simulink model "LQI"  (R2024a)
settings: Solver=VariableStepAuto  StartTime=0.0  StopTime=2.5  RelTol=1e-3
values from neighbouring files (symbols this model uses):
  A = [A11 A12 A13 A14; A21 A22 A23 A24; A31 A32 A33 A34; A41 A42 A43 A44]    [FurutaLineal.m]    (also in ModeloFuruta.m = [0      0       1       0)
  B = [B11 B12; B21 B22; B31 B32; B41 B42]    [FurutaLineal.m]    (also in ModeloFuruta.m = [0)
  D = [2*I_x*block.ContStates.Data(4)*cos(block.ContStates.Data(2))*sin(block.ContStates.Data(2)), -C_z*M_2*l_bi*sin(block.ContStates.Data(2))*block.ContStates.Data(4); -I_x*block.ContStates.Data(3)*cos(block.ContStates.Data(2))*sin(block.ContStates.Data(2)), 0]    [FurutanolinealSLV2.m]
  K = 1.29    [FurutanolinealSLV2.m]
undefined symbols (not defined in the file or in its folder): A1, B1, C, C1, D1, K1
settings Model: Creator=PC  LastModifiedBy=PC
settings SolverCC: MaxConsecutiveMinStep=100
settings RTWCC: GPUComputeCapability=3.5

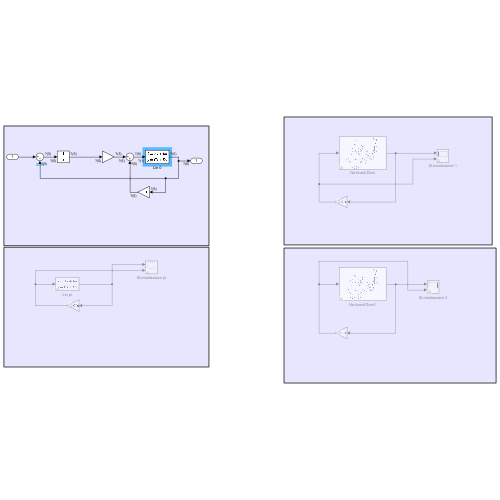
[thumbnail: Simulink's stored preview of the top-level diagram]
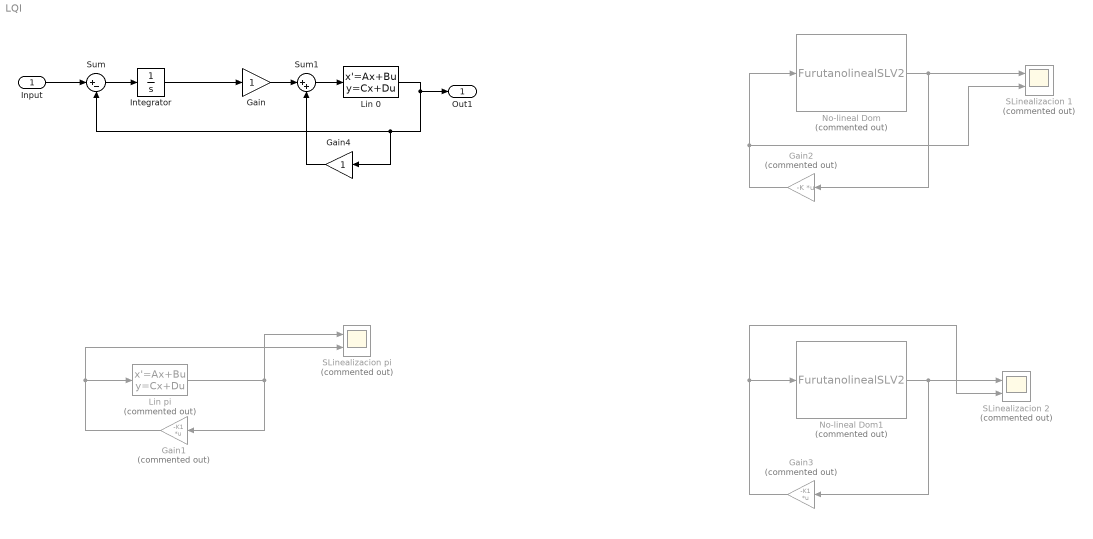
== system LQI ==
  Input : Inport
  Gain : Gain
  Gain1 : Gain  Commented=on  Gain=-K1  Multiplication=Matrix(K*u)
  Gain2 : Gain  Commented=on  Gain=-K  Multiplication=Matrix(K*u)
  Gain3 : Gain  Commented=on  Gain=-K1  Multiplication=Matrix(K*u)
  Gain4 : Gain
  Integrator : Integrator
  Lin 0 : StateSpace  A=A  B=B  C=C  D=D  InitialCondition=[0;0;0;0;0]  ParameterTunability=Unconstrained  AllowTunableDMatrix=on
  Lin pi : StateSpace  Commented=on  A=A1  B=B1  C=C1  D=D1  InitialCondition=[0;pi;0;0;0]  ParameterTunability=Unconstrained  AllowTunableDMatrix=on
  No-lineal Dom : M-S-Function  Commented=on  FunctionName=FurutanolinealSLV2  mask{Xi=0, g=0, J=0, M_2=0, l_bi=0, C_x=0, C_z=0, I_x=0, I_z=0}
      mask prompts: Xi "Parametros iniciales (Xi)"
      mask Display: image('mascara2.png');
  No-lineal Dom1 : M-S-Function  Commented=on  FunctionName=FurutanolinealSLV2  mask{Xi=0, g=0, J=0, M_2=0, l_bi=0, C_x=0, C_z=0, I_x=0, I_z=0}
      mask prompts: Xi "Parametros iniciales (Xi)"
      mask Display: image('mascara2.png');
  SLinealizacion 1 : Scope  Commented=on  NumInputPorts=2
  SLinealizacion 2 : Scope  Commented=on  NumInputPorts=2
  SLinealizacion pi : Scope  Commented=on  NumInputPorts=2
  Sum : Sum  Inputs=|+-
  Sum1 : Sum  Inputs=|++
  Out1 : Outport
  wires:
  Lin pi/1 -> Gain1/1, SLinealizacion pi/1
  Gain1/1 -> SLinealizacion pi/2, Lin pi/1
  No-lineal Dom/1 -> Gain2/1, SLinealizacion 1/1
  Gain2/1 -> No-lineal Dom/1, SLinealizacion 1/2
  Gain3/1 -> No-lineal Dom1/1, SLinealizacion 2/2
  No-lineal Dom1/1 -> Gain3/1, SLinealizacion 2/1
  Lin 0/1 -> Out1/1, Gain4/1, Sum/2
  Sum/1 -> Integrator/1
  Input/1 -> Sum/1
  Integrator/1 -> Gain/1
  Gain/1 -> Sum1/1
  Gain4/1 -> Sum1/2
  Sum1/1 -> Lin 0/1
